simulink model "cv_model"  (R2023a)
settings: Solver=ode23t  StartTime=0  StopTime=400  FixedStep=0.0005  MaxStep=.01  RelTol=1e-4
model workspace (MAT data in the model file):
  test = 0
values from neighbouring files (symbols this model uses):
  A_cheb_09_1 = [-9.45889157397 1 0 0 0 0 0 0 0 -116.684730988 0 1 ... (81 elements, 9x9)]    [input_reflex_filters.mat]
  B_cheb_09_1 = [1 0 0 0 0 0 0 0 0]    [input_reflex_filters.mat]
  C_cheb_09_1 = [0 0 0 0 0 0 0 0 151338.279895]    [input_reflex_filters.mat]
libraries: SignalEditorBlockLib x4, simulink_extras x2
(part 1 of 3)
settings Model: ExtModeTrigMode=oneshot  Creator=samar  LastModifiedBy=Rich
settings SolverCC: AlgebraicLoopSolver=TrustRegion
settings DataIOCC: SaveFormat=Array  SignalLoggingSaveFormat=ModelDataLogs  ReturnWorkspaceOutputs=off  SignalLoggingName=sigsOut
settings OptimizationCC: BooleanDataType=off  InitFltsAndDblsToZero=on  LifeSpan=inf
settings DebuggingCC: ConsistencyChecking=warning  SaveWithParameterizedLinksMsg=none  UnderspecifiedInitializationDetection=Classic  MergeDetectMultiDrivingBlocksExec=none  SignalResolutionControl=TryResolveAllWithWarning  MultiTaskDSMMsg=warning  MultiTaskCondExecSysMsg=none  FcnCallInpInsideContextMsg=warning  SFUnexpectedBacktrackingDiag=warning  SFNoUnconditionalDefaultTransitionDiag=warning  SFExecutionAtInitializationDiag=none  ArithmeticOperatorsInVariantConditions=warning
settings HardwareCC: ProdBitPerPointer=32  ProdBitPerSizeT=32  ProdBitPerPtrDiffT=32  ProdLargestAtomicFloat=None  ProdIntDivRoundTo=Undefined  ProdEndianess=Unspecified  ProdWordSize=32  ProdHWDeviceType=32-bit Generic  TargetUnknown=on
settings ModelReferenceCC: EnableRefExpFcnMdlSchedulingChecks=on  PropagateSignalLabelsOutOfModel=off
settings SFSimCC: SimUseLocalCustomCode=off  CustomCodeUndefinedFunction=UseInterfaceOnly
settings RTWCC: TemplateMakefile=grt_unix.tmf  RTWUseLocalCustomCode=off  DLArmComputeVersion=19.05
settings CodeAppCC: StateflowObjectComments=on
settings GRTTargetCC: TargetFcnLib=ansi_tfl_tmw.mat  TargetLangStandard=C89/C90 (ANSI)  ModelReferenceCompliant=off  CombineOutputUpdateFcns=off  MatFileLogging=off  GRTInterface=on
settings ConfigComp: CovMetricSettings=dw  CovSaveCumulativeToWorkspaceVar=on  CovSaveSingleToWorkspaceVar=on  CovExternalEMLEnable=off  CovSFcnEnable=off

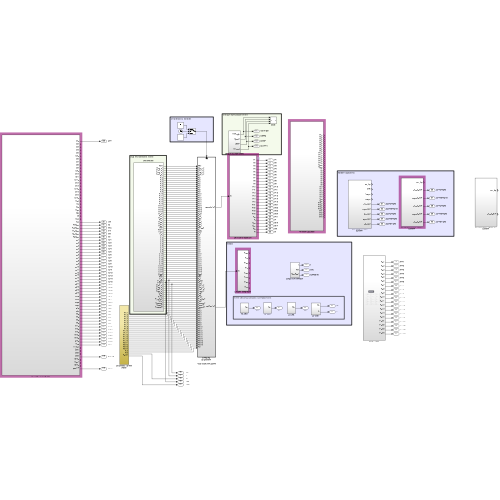
[thumbnail: Simulink's stored preview of the top-level diagram]
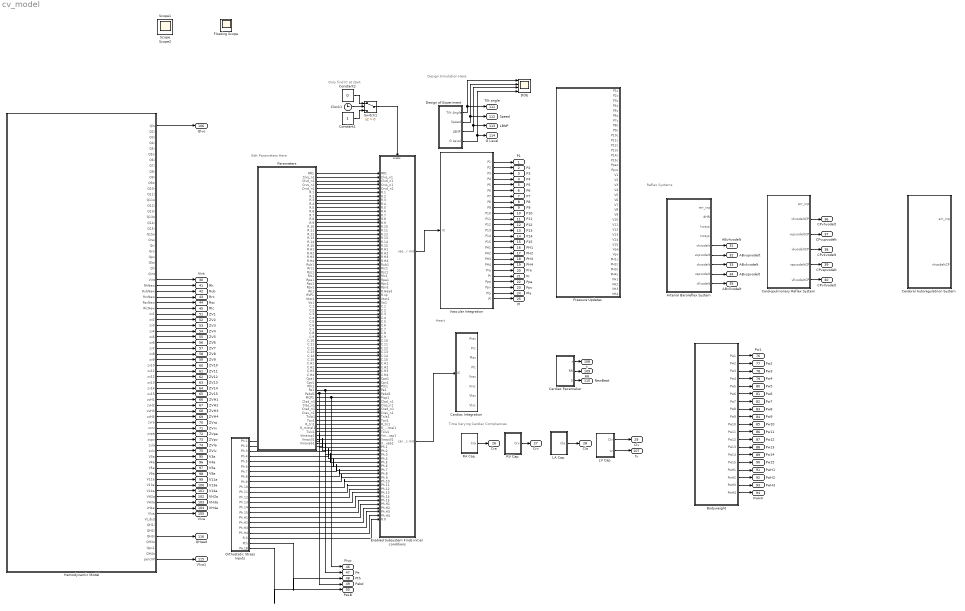
== system cv_model ==
  note: Design Simulation Here
  note: Edit Parameters Here
  note: Reflex Systems
  note: Heart
  note: Time Varying Cardiac Compliances
  note: Only find IC at start
  Arterial Baroreflex System : Subsystem
  Bodyweight : Subsystem
  Cardiac Integration : Subsystem
  Cardiac Pacemaker : Subsystem
  Cardiopulmonary Reflex System : Subsystem
  Cerebral Autoregulatrion System : Subsystem
  Clock1 : Clock
  Constant1 : Constant
  Constant2 : Constant  Value=0
  DOE : Scope  NumInputPorts=4
  Design of Experiment : Subsystem
  Enabled Subsystem Finds initial conditions : Subsystem  TreatAsAtomicUnit=on
  Hemodynamic Model : Subsystem
  LA Cap. : Subsystem
  LV Cap. : Subsystem
  Orthostatic Stress Inputs : Subsystem
  Parameters : Subsystem
  Pressure Updates : Subsystem
  RA Cap. : Subsystem
  RV Cap. : Subsystem
  Switch1 : Switch  Criteria=u2 > Threshold
  Vascular Integration : Subsystem
  P1 : Outport
  P2 : Outport  Port=2
  P3 : Outport  Port=3
  P4 : Outport  Port=4
  P5 : Outport  Port=5
  P6 : Outport  Port=6
  P7 : Outport  Port=7
  P8 : Outport  Port=8
  P9 : Outport  Port=9
  P10 : Outport  Port=10
  P11 : Outport  Port=11
  P12 : Outport  Port=12
  P13 : Outport  Port=13
  P14 : Outport  Port=14
  P15 : Outport  Port=15
  PH1 : Outport  Port=16
  PH2 : Outport  Port=17
  PH3 : Outport  Port=18
  PH4 : Outport  Port=19
  Pra : Outport  Port=20
  Pr : Outport  Port=21
  Ppa : Outport  Port=22
  Ppv : Outport  Port=23
  Pla : Outport  Port=24
  Pl : Outport  Port=25
  Cra : Outport  Port=26
  Crv : Outport  Port=27
  Cla : Outport  Port=28
  Clv : Outport  Port=29
  Vint : Outport  Port=30
  ABvhvodelt : Outport  Port=31
  ABvupvodelt : Outport  Port=32
  ABvkvodelt : Outport  Port=33
  ABvspvodelt : Outport  Port=34
  ABvllvodelt : Outport  Port=35
  CPvhvodelt : Outport  Port=36
  CPvupvodelt : Outport  Port=37
  CPvkvodelt : Outport  Port=38
  CPvspvodelt : Outport  Port=39
  CPvllvodelt : Outport  Port=40
  Rh : Outport  Port=41
  Rub : Outport  Port=42
  Rrc : Outport  Port=43
  Rsc : Outport  Port=44
  Rlc : Outport  Port=45
  Picp : Outport  Port=46
  Pe : Outport  Port=47
  Pth : Outport  Port=48
  Pabd : Outport  Port=49
  PeLB : Outport  Port=50
  ZV1 : Outport  Port=51
  ZV2 : Outport  Port=52
  ZV3 : Outport  Port=53
  ZV4 : Outport  Port=54
  ZV5 : Outport  Port=55
  ZV6 : Outport  Port=56
  ZV7 : Outport  Port=57
  ZV8 : Outport  Port=58
  ZV9 : Outport  Port=59
  ZV10 : Outport  Port=60
  ZV11 : Outport  Port=61
  ZV12 : Outport  Port=62
  ZV13 : Outport  Port=63
  ZV14 : Outport  Port=64
  ZV15 : Outport  Port=65
  ZVH1 : Outport  Port=66
  ZVH2 : Outport  Port=67
  ZVH3 : Outport  Port=68
  ZVH4 : Outport  Port=69
  ZVra : Outport  Port=70
  ZVrv : Outport  Port=71
  ZVpa : Outport  Port=72
  ZVpv : Outport  Port=73
  ZVla : Outport  Port=74
  ZVlv : Outport  Port=75
  Pw1 : Outport  Port=76
  Pw2 : Outport  Port=77
  Pw3 : Outport  Port=78
  Pw4 : Outport  Port=79
  Pw5 : Outport  Port=80
  Pw6 : Outport  Port=81
  Pw7 : Outport  Port=82
  Pw8 : Outport  Port=83
  Pw9 : Outport  Port=84
  Pw10 : Outport  Port=85
  Pw11 : Outport  Port=86
  Pw12 : Outport  Port=87
  Pw13 : Outport  Port=88
  Pw14 : Outport  Port=89
  Pw15 : Outport  Port=90
  PwH1 : Outport  Port=91
  PwH2 : Outport  Port=92
  PwH3 : Outport  Port=93
  PwH4 : Outport  Port=94
  V3a : Outport  Port=95
  V4a : Outport  Port=96
  V5a : Outport  Port=97
  V9a : Outport  Port=98
  V11a : Outport  Port=99
  V13a : Outport  Port=100
  V14a : Outport  Port=101
  VH2a : Outport  Port=102
  VH3a : Outport  Port=103
  VH4a : Outport  Port=104
  Vlva : Outport  Port=105
  Qlvo : Outport  Port=106
  tv : Outport  Port=107
  t : Outport  Port=108
  RR : Outport  Port=109
  NewBeat : Outport  Port=110
  Tilt angle : Outport  Port=111
  Speed : Outport  Port=112
  LBNP : Outport  Port=113
  G Level : Outport  Port=114
  Vlva1 : Outport  Port=115
  QHead : Outport  Port=116
  Floating Scope : Scope
  Scope : Scope
  Scope1 : Scope
  Scope2 : Scope
  wires:
  Enabled Subsystem Finds initial conditions/2(cardiac init) -> Cardiac Integration/1(IC)
  Enabled Subsystem Finds initial conditions/1(vascular init) -> Vascular Integration/1(IC)
  Constant2/1 -> Switch1/1
  Clock1/1 -> Switch1/2
  Constant1/1 -> Switch1/3
  Vascular Integration/25(Pl) -> Pl/1
  Vascular Integration/21(Pr) -> Pr/1
  Vascular Integration/22(Ppa) -> Ppa/1
  Vascular Integration/23(Ppv) -> Ppv/1
  Vascular Integration/1(P1) -> P1/1
  Vascular Integration/2(P2) -> P2/1
  Vascular Integration/3(P3) -> P3/1
  Vascular Integration/4(P4) -> P4/1
  Vascular Integration/5(P5) -> P5/1
  Vascular Integration/6(P6) -> P6/1
  Vascular Integration/7(P7) -> P7/1
  Vascular Integration/8(P8) -> P8/1
  Vascular Integration/9(P9) -> P9/1
  Vascular Integration/10(P10) -> P10/1
  Vascular Integration/11(P11) -> P11/1
  Vascular Integration/12(P12) -> P12/1
  Vascular Integration/13(P13) -> P13/1
  Vascular Integration/14(P14) -> P14/1
  Vascular Integration/15(P15) -> P15/1
  Arterial Baroreflex System/8(vspvodelt) -> ABvspvodelt/1
  Arterial Baroreflex System/6(vupvodelt) -> ABvupvodelt/1
  Cardiopulmonary Reflex System/5(vspvodeltCP) -> CPvspvodelt/1
  Cardiopulmonary Reflex System/4(vkvodeltCP) -> CPvkvodelt/1
  Cardiopulmonary Reflex System/6(vllvodeltCP) -> CPvllvodelt/1
  RA Cap./1(Cra) -> Cra/1
  LA Cap./1(Cla) -> Cla/1
  Cardiac Pacemaker/1(t) -> t/1
  LV Cap./1(Clv) -> Clv/1
  LV Cap./2(tv) -> tv/1
  RV Cap./1(Crv) -> Crv/1
  Vascular Integration/20(Pra) -> Pra/1
  Vascular Integration/24(Pla) -> Pla/1
  Arterial Baroreflex System/7(vkvodelt) -> ABvkvodelt/1
  Arterial Baroreflex System/9(vllvodelt) -> ABvllvodelt/1
  Cardiopulmonary Reflex System/3(vupvodeltCP) -> CPvupvodelt/1
  Orthostatic Stress Inputs/21(Pth) -> Pth/1
  Cardiac Pacemaker/2(RR) -> RR/1
  Cardiac Pacemaker/3(NewBeat) -> NewBeat/1
  Orthostatic Stress Inputs/22(Pe.LB) -> PeLB/1
  Hemodynamic Model/63(V11a) -> V11a/1
  Hemodynamic Model/33(RlcNew) -> Rlc/1
  Hemodynamic Model/62(V9a) -> V9a/1
  Hemodynamic Model/31(RrcNew) -> Rrc/1
  Hemodynamic Model/59(V3a) -> V3a/1
  Hemodynamic Model/32(RscNew) -> Rsc/1
  Hemodynamic Model/65(V14a) -> V14a/1
  Hemodynamic Model/69(Vlva) -> Vlva/1
  Hemodynamic Model/60(V4a) -> V4a/1
  Hemodynamic Model/30(RubNew) -> Rub/1
  Hemodynamic Model/61(V5a) -> V5a/1
  Design of Experiment/3(LBNP) -> DOE/3, LBNP/1
  Design of Experiment/1(Tilt Angle) -> Tilt angle/1, DOE/1
  Hemodynamic Model/28(Vint) -> Vint/1
  Design of Experiment/4(G Level) -> DOE/4, G Level/1
  Design of Experiment/2(Speed) -> DOE/2, Speed/1
  Parameters/59(Pabd1) -> Enabled Subsystem Finds initial conditions/59(Pabd1), Pabd/1
  Parameters/61(Clad_n1) -> Enabled Subsystem Finds initial conditions/61(Clad_n1)
  Parameters/62(Clas_n1) -> Enabled Subsystem Finds initial conditions/62(Clas_n1)
  Parameters/63(Crad_n1) -> Enabled Subsystem Finds initial conditions/63(Crad_n1)
  Parameters/64(Cras_n1) -> Enabled Subsystem Finds initial conditions/64(Cras_n1)
  Parameters/65(Tsla1) -> Enabled Subsystem Finds initial conditions/65(Tsla1)
  Parameters/66(Tav1) -> Enabled Subsystem Finds initial conditions/66(Tav1)
  Parameters/67(R_tri1) -> Enabled Subsystem Finds initial conditions/67(R_tri1)
  Parameters/68(R_mitral1) -> Enabled Subsystem Finds initial conditions/68(R_mitral1)
  Parameters/69(Tslv1) -> Enabled Subsystem Finds initial conditions/69(Tslv1)
  Parameters/70(Vmaxsp1) -> Enabled Subsystem Finds initial conditions/70(Vmaxsp1)
  Parameters/71(Vmaxll1) -> Enabled Subsystem Finds initial conditions/71(Vmaxll1)
  Parameters/72(Vmaxab1) -> Enabled Subsystem Finds initial conditions/72(Vmaxab1)
  Orthostatic Stress Inputs/1(Ph.1) -> Enabled Subsystem Finds initial conditions/73(Ph.1)
  Orthostatic Stress Inputs/2(Ph.2) -> Enabled Subsystem Finds initial conditions/74(Ph.2)
  Orthostatic Stress Inputs/3(Ph.3) -> Enabled Subsystem Finds initial conditions/75(Ph.3)
  Orthostatic Stress Inputs/4(Ph.4) -> Enabled Subsystem Finds initial conditions/76(Ph.4)
  Orthostatic Stress Inputs/5(Ph.5) -> Enabled Subsystem Finds initial conditions/77(Ph.5)
  Orthostatic Stress Inputs/6(Ph.6) -> Enabled Subsystem Finds initial conditions/78(Ph.6)
  Orthostatic Stress Inputs/7(Ph.7) -> Enabled Subsystem Finds initial conditions/79(Ph.7)
  Orthostatic Stress Inputs/8(Ph.8) -> Enabled Subsystem Finds initial conditions/80(Ph.8)
  Orthostatic Stress Inputs/9(Ph.9) -> Enabled Subsystem Finds initial conditions/81(Ph.9)
  Orthostatic Stress Inputs/10(Ph.10) -> Enabled Subsystem Finds initial conditions/82(Ph.10)
  Orthostatic Stress Inputs/11(Ph.11) -> Enabled Subsystem Finds initial conditions/83(Ph.11)
  Orthostatic Stress Inputs/12(Ph.12) -> Enabled Subsystem Finds initial conditions/84(Ph.12)
  Orthostatic Stress Inputs/13(Ph.13) -> Enabled Subsystem Finds initial conditions/85(Ph.13)
  Orthostatic Stress Inputs/14(Ph.14) -> Enabled Subsystem Finds initial conditions/86(Ph.14)
  Orthostatic Stress Inputs/15(Ph.15) -> Enabled Subsystem Finds initial conditions/87(Ph.15)
  Orthostatic Stress Inputs/20(R.0) -> Enabled Subsystem Finds initial conditions/92(R.0)
  Parameters/1(RR1) -> Enabled Subsystem Finds initial conditions/1(RR1)
  Parameters/2(Clvs_n1) -> Enabled Subsystem Finds initial conditions/2(Clvs_n1)
  Parameters/3(Clvd_n1) -> Enabled Subsystem Finds initial conditions/3(Clvd_n1)
  Parameters/4(Crvs_n1) -> Enabled Subsystem Finds initial conditions/4(Crvs_n1)
  Parameters/5(Crvd_n1) -> Enabled Subsystem Finds initial conditions/5(Crvd_n1)
  Parameters/6(R.1) -> Enabled Subsystem Finds initial conditions/6(R.1)
  Parameters/7(R.2) -> Enabled Subsystem Finds initial conditions/7(R.2)
  Parameters/8(R.3) -> Enabled Subsystem Finds initial conditions/8(R.3)
  Parameters/9(R.4) -> Enabled Subsystem Finds initial conditions/9(R.4)
  Parameters/10(R.5) -> Enabled Subsystem Finds initial conditions/10(R.5)
  Parameters/11(R.6) -> Enabled Subsystem Finds initial conditions/11(R.6)
  Parameters/12(R.7) -> Enabled Subsystem Finds initial conditions/12(R.7)
  Parameters/13(R.8) -> Enabled Subsystem Finds initial conditions/13(R.8)
  Parameters/14(R.9) -> Enabled Subsystem Finds initial conditions/14(R.9)
  Parameters/15(R.10) -> Enabled Subsystem Finds initial conditions/15(R.10)
  Parameters/16(R.11) -> Enabled Subsystem Finds initial conditions/16(R.11)
  Parameters/17(R.12) -> Enabled Subsystem Finds initial conditions/17(R.12)
  Parameters/18(R.13) -> Enabled Subsystem Finds initial conditions/18(R.13)
  Parameters/19(R.14) -> Enabled Subsystem Finds initial conditions/19(R.14)
  Parameters/20(R.15) -> Enabled Subsystem Finds initial conditions/20(R.15)
  Parameters/25(Rub1) -> Enabled Subsystem Finds initial conditions/25(Rub1)
  Parameters/26(Rrc1) -> Enabled Subsystem Finds initial conditions/26(Rrc1)
  Parameters/27(Rsc1) -> Enabled Subsystem Finds initial conditions/27(Rsc1)
  Parameters/28(Rlc1) -> Enabled Subsystem Finds initial conditions/28(Rlc1)
  Parameters/29(Rpa1) -> Enabled Subsystem Finds initial conditions/29(Rpa1)
  Parameters/30(Rpc1) -> Enabled Subsystem Finds initial conditions/30(Rpc1)
  Parameters/31(Rpv1) -> Enabled Subsystem Finds initial conditions/31(Rpv1)
  Parameters/34(Vtot1) -> Enabled Subsystem Finds initial conditions/34(Vtot1)
  Parameters/35(Vo1) -> Enabled Subsystem Finds initial conditions/35(Vo1)
  Parameters/36(C.1) -> Enabled Subsystem Finds initial conditions/36(C.1)
  Parameters/37(C.2) -> Enabled Subsystem Finds initial conditions/37(C.2)
  Parameters/38(C.3) -> Enabled Subsystem Finds initial conditions/38(C.3)
  Parameters/39(C.4) -> Enabled Subsystem Finds initial conditions/39(C.4)
  Parameters/40(C.5) -> Enabled Subsystem Finds initial conditions/40(C.5)
  Parameters/41(C.6) -> Enabled Subsystem Finds initial conditions/41(C.6)
  Parameters/42(C.7) -> Enabled Subsystem Finds initial conditions/42(C.7)
  Parameters/43(C.8) -> Enabled Subsystem Finds initial conditions/43(C.8)
  Parameters/44(C.9) -> Enabled Subsystem Finds initial conditions/44(C.9)
  Parameters/45(C.10) -> Enabled Subsystem Finds initial conditions/45(C.10)
  Parameters/46(C.11) -> Enabled Subsystem Finds initial conditions/46(C.11)
  Parameters/47(C.12) -> Enabled Subsystem Finds initial conditions/47(C.12)
  Parameters/48(C.13) -> Enabled Subsystem Finds initial conditions/48(C.13)
  Parameters/49(C.14) -> Enabled Subsystem Finds initial conditions/49(C.14)
  Parameters/50(C.15) -> Enabled Subsystem Finds initial conditions/50(C.15)
  Parameters/55(Cpa1) -> Enabled Subsystem Finds initial conditions/55(Cpa1)
  Parameters/56(Cpv1) -> Enabled Subsystem Finds initial conditions/56(Cpv1)
  Parameters/57(Pth1) -> Enabled Subsystem Finds initial conditions/57(Pth1)
  Hemodynamic Model/34(zv1) -> ZV1/1
  Hemodynamic Model/35(zv2) -> ZV2/1
  Hemodynamic Model/36(zv3) -> ZV3/1
  Hemodynamic Model/37(zv4) -> ZV4/1
  Hemodynamic Model/38(zv5) -> ZV5/1
  Hemodynamic Model/39(zv6) -> ZV6/1
  Hemodynamic Model/40(zv7) -> ZV7/1
  Hemodynamic Model/41(zv8) -> ZV8/1
  Hemodynamic Model/42(zv9) -> ZV9/1
  Hemodynamic Model/43(zv10) -> ZV10/1
  Hemodynamic Model/44(zv11) -> ZV11/1
  Hemodynamic Model/45(zv12) -> ZV12/1
  Hemodynamic Model/46(zv13) -> ZV13/1
  Hemodynamic Model/47(zv14) -> ZV14/1
  Hemodynamic Model/48(zv15) -> ZV15/1
  Hemodynamic Model/53(zvra) -> ZVra/1
  Hemodynamic Model/54(zvrv) -> ZVrv/1
  Hemodynamic Model/55(zvpa) -> ZVpa/1
  Hemodynamic Model/56(zvpv) -> ZVpv/1
  Hemodynamic Model/57(zvla) -> ZVla/1
  Hemodynamic Model/58(zvlv) -> ZVlv/1
  Hemodynamic Model/64(V13a) -> V13a/1
  Hemodynamic Model/1(Qlo) -> Qlvo/1
  Switch1/1 -> Enabled Subsystem Finds initial conditions/Enable
  Parameters/21(R.H1) -> Enabled Subsystem Finds initial conditions/21(R.H1)
  Parameters/22(R.H2) -> Enabled Subsystem Finds initial conditions/22(R.H2)
  Parameters/23(R.H3) -> Enabled Subsystem Finds initial conditions/23(R.H3)
  Parameters/24(R.H4) -> Enabled Subsystem Finds initial conditions/24(R.H4)
  Parameters/32(Rh1) -> Enabled Subsystem Finds initial conditions/32(R.Head)
  Parameters/33(RVP1) -> Enabled Subsystem Finds initial conditions/33(R.vp)
  Parameters/51(C.H1) -> Enabled Subsystem Finds initial conditions/51(C.H1)
  Parameters/52(C.H2) -> Enabled Subsystem Finds initial conditions/52(C.H2)
  Parameters/53(C.H3) -> Enabled Subsystem Finds initial conditions/53(C.H3)
  Parameters/54(C.H4) -> Enabled Subsystem Finds initial conditions/54(C.H4)
  Parameters/60(PICP1) -> Enabled Subsystem Finds initial conditions/60(Picp1), Picp/1
  Orthostatic Stress Inputs/16(Ph.H1) -> Enabled Subsystem Finds initial conditions/88(Ph.H1)
  Orthostatic Stress Inputs/17(Ph.H2) -> Enabled Subsystem Finds initial conditions/89(Ph.H2)
  Orthostatic Stress Inputs/18(Ph.H3) -> Enabled Subsystem Finds initial conditions/90(Ph.H3)
  Orthostatic Stress Inputs/19(Ph.H4) -> Enabled Subsystem Finds initial conditions/91(Ph.H4)
  Vascular Integration/16(PH1) -> PH1/1
  Vascular Integration/17(PH2) -> PH2/1
  Vascular Integration/18(PH3) -> PH3/1
  Vascular Integration/19(PH4) -> PH4/1
  Arterial Baroreflex System/5(vhvodelt) -> ABvhvodelt/1
  Cardiopulmonary Reflex System/2(vhvodeltCP) -> CPvhvodelt/1
  Hemodynamic Model/29(RhNew) -> Rh/1
  Hemodynamic Model/49(zvH1) -> ZVH1/1
  Hemodynamic Model/50(zvH2) -> ZVH2/1
  Hemodynamic Model/51(zvH3) -> ZVH3/1
  Hemodynamic Model/52(zvH4) -> ZVH4/1
  Hemodynamic Model/66(VH2a) -> VH2a/1
  Hemodynamic Model/67(VH3a) -> VH3a/1
  Hemodynamic Model/68(vH4a) -> VH4a/1
  Parameters/58(Pe1) -> Enabled Subsystem Finds initial conditions/58(Pe1), Pe/1
  Bodyweight/1(Pw1) -> Pw1/1
  Bodyweight/2(Pw2) -> Pw2/1
  Bodyweight/3(Pw3) -> Pw3/1
  Bodyweight/4(Pw4) -> Pw4/1
  Bodyweight/5(Pw5) -> Pw5/1
  Bodyweight/6(Pw6) -> Pw6/1
  Bodyweight/7(Pw7) -> Pw7/1
  Bodyweight/8(Pw8) -> Pw8/1
  Bodyweight/9(Pw9) -> Pw9/1
  Bodyweight/10(Pw10) -> Pw10/1
  Bodyweight/11(Pw11) -> Pw11/1
  Bodyweight/12(Pw12) -> Pw12/1
  Bodyweight/13(Pw13) -> Pw13/1
  Bodyweight/14(Pw14) -> Pw14/1
  Bodyweight/15(Pw15) -> Pw15/1
  Bodyweight/16(PwH1) -> PwH1/1
  Bodyweight/17(PwH2) -> PwH2/1
  Bodyweight/18(PwH3) -> PwH3/1
  Bodyweight/19(PwH4) -> PwH4/1
  Hemodynamic Model/77(percVP) -> Vlva1/1
  Hemodynamic Model/73(QH3i) -> QHead/1

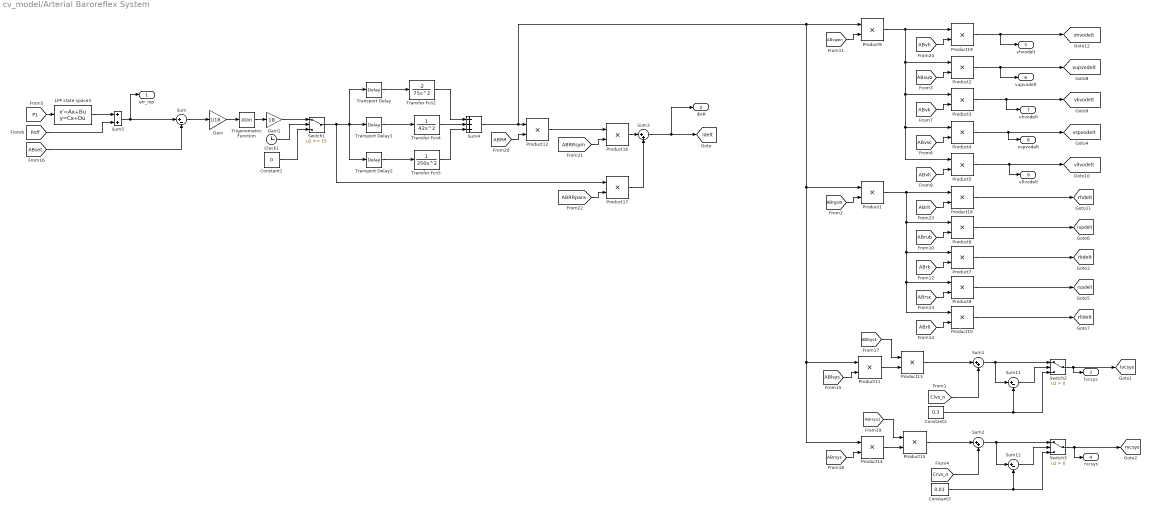
== system cv_model/Arterial Baroreflex System ==
  Clock1 : Clock
  Constant1 : Constant  Value=0
  Constant2 : Constant  Value=0.3
  Constant3 : Constant  Value=0.01
  Gain : Gain  Gain=1/18  SaturateOnIntegerOverflow=on  OutDataTypeStr=Inherit: Same as input  ParamDataTypeStr=Inherit: Same as input
  Gain1 : Gain  Gain=18  SaturateOnIntegerOverflow=on  OutDataTypeStr=Inherit: Same as input  ParamDataTypeStr=Inherit: Same as input
  LPF state space3 : StateSpace  A=A_cheb_09_1  B=B_cheb_09_1  C=C_cheb_09_1  D=0  InitialCondition=[0 0 0 0 0 0 0 0 91/C_cheb_09_1(9)]
  Product{1..19} (19 alike) : Product  Inputs=**  SaturateOnIntegerOverflow=on  OutDataTypeStr=Inherit: Same as first input
  Sum : Sum  Inputs=|+-  InputSameDT=on  SaturateOnIntegerOverflow=on  OutDataTypeStr=Inherit: Same as first input
  Sum1 : Sum  Inputs=|++  InputSameDT=on  SaturateOnIntegerOverflow=on  OutDataTypeStr=Inherit: Same as first input
  Sum11 : Sum  Inputs=|+-  InputSameDT=on  SaturateOnIntegerOverflow=on  OutDataTypeStr=Inherit: Same as first input
  Sum12 : Sum  Inputs=|+-  InputSameDT=on  SaturateOnIntegerOverflow=on  OutDataTypeStr=Inherit: Same as first input
  Sum2 : Sum  Inputs=|++  InputSameDT=on  SaturateOnIntegerOverflow=on  OutDataTypeStr=Inherit: Same as first input
  Sum3 : Sum  Inputs=|++  InputSameDT=on  SaturateOnIntegerOverflow=on  OutDataTypeStr=Inherit: Same as first input
  Sum4 : Sum  Inputs=+++  InputSameDT=on  SaturateOnIntegerOverflow=on  OutDataTypeStr=Inherit: Same as first input
  Sum5 : Sum  InputSameDT=on  SaturateOnIntegerOverflow=on  OutDataTypeStr=Inherit: Same as first input
  Switch1 : Switch  Threshold=15
  Switch2 : Switch  Criteria=u2 > Threshold
  Switch3 : Switch  Criteria=u2 > Threshold
  Transfer Fcn2 : TransferFcn  Numerator=-2  Denominator=[75 0 0]
  Transfer Fcn4 : TransferFcn  Numerator=1  Denominator=[42 0 0 ]
  Transfer Fcn5 : TransferFcn  Numerator=1  Denominator=[350 0 0 ]
  Transport Delay : TransportDelay  DelayTime=5
  Transport Delay1 : TransportDelay  DelayTime=2
  Transport Delay2 : TransportDelay  DelayTime=30  BufferSize=6144
  Trigonometric Function : Trigonometry  Operator=atan
  err_inp : Outport
  dHR : Outport  Port=2
  lvcsys : Outport  Port=3
  rvcsys : Outport  Port=4
  vhvodelt : Outport  Port=5
  vupvodelt : Outport  Port=6
  vkvodelt : Outport  Port=7
  vspvodelt : Outport  Port=8
  vllvodelt : Outport  Port=9
  tag scope: idelt=global, lvcsys=global, rhdelt=global, rkdelt=global, rlldelt=global, rspdelt=global, rupdelt=global, rvcsys=global, vhvodelt=global, vkvodelt=global, vllvodelt=global, vspvodelt=global, vupvodelt=global
  wires:
  Sum/1 -> Gain/1
  Product15/1 -> Sum2/1
  Product13/1 -> Sum1/1
  Sum1/1 -> Sum11/1, Switch2/1
  Product7/1 -> [rkdelt]
  Product4/1 -> [vspvodelt], vspvodelt/1
  [Crvs_n] -> Sum2/2
  [Clvs_n] -> Sum1/2
  Trigonometric Function/1 -> Gain1/1
  Product10/1 -> [rlldelt]
  Product6/1 -> [rupdelt]
  Product8/1 -> [rspdelt]
  Product2/1 -> vupvodelt/1, [vupvodelt]
  Product3/1 -> vkvodelt/1, [vkvodelt]
  Product5/1 -> vllvodelt/1, [vllvodelt]
  Product9/1 -> Product19/1, Product2/1, Product3/1, Product4/1, Product5/1
  Product1/1 -> Product18/1, Product6/1, Product7/1, Product8/1, Product10/1
  Sum4/1 -> Product12/1, Product9/1, Product14/1, Product11/1, Product1/1
  Gain1/1 -> Switch1/1
  Product16/1 -> Sum3/1
  Sum3/1 -> [idelt], dHR/1
  Product17/1 -> Sum3/2
  Clock1/1 -> Switch1/2
  Constant1/1 -> Switch1/3
  Switch1/1 -> Product17/1, Transport Delay1/1, Transport Delay/1, Transport Delay2/1
  Gain/1 -> Trigonometric Function/1
  Sum5/1 -> err_inp/1, Sum/1
  Sum11/1 -> Switch2/2
  Constant2/1 -> Switch2/3, Sum11/2
  Switch2/1 -> [lvcsys], lvcsys/1
  Sum2/1 -> Switch3/1, Sum12/1
  Sum12/1 -> Switch3/2
  Constant3/1 -> Switch3/3, Sum12/2
  Switch3/1 -> [rvcsys], rvcsys/1
  [P1] -> LPF state space3/1
  Transport Delay/1 -> Transfer Fcn2/1
  Transport Delay1/1 -> Transfer Fcn4/1
  Transport Delay2/1 -> Transfer Fcn5/1
  Transfer Fcn2/1 -> Sum4/1
  Transfer Fcn4/1 -> Sum4/2
  Transfer Fcn5/1 -> Sum4/3
  LPF state space3/1 -> Sum5/1
  [Poff] -> Sum5/2
  [ABset] -> Sum/2
  [ABvgain] -> Product9/2
  [ABrgain] -> Product1/2
  [ABvub] -> Product2/2
  [ABvk] -> Product3/2
  [ABvsc] -> Product4/2
  [ABvll] -> Product5/2
  [ABrub] -> Product6/2
  [ABrk] -> Product7/2
  [ABrsc] -> Product8/2
  [ABrll] -> Product10/2
  [ABlsys] -> Product11/2
  Product11/1 -> Product13/2
  [ABlsys1] -> Product13/1
  [ABrsys1] -> Product15/1
  [ABrsys] -> Product14/2
  Product14/1 -> Product15/2
  [ABRR] -> Product12/2
  [ABRRsym] -> Product16/2
  Product12/1 -> Product16/1
  [ABRRpara] -> Product17/2
  [ABrh] -> Product18/2
  Product18/1 -> [rhdelt]
  Product19/1 -> vhvodelt/1, [vhvodelt]
  [ABvh] -> Product19/2

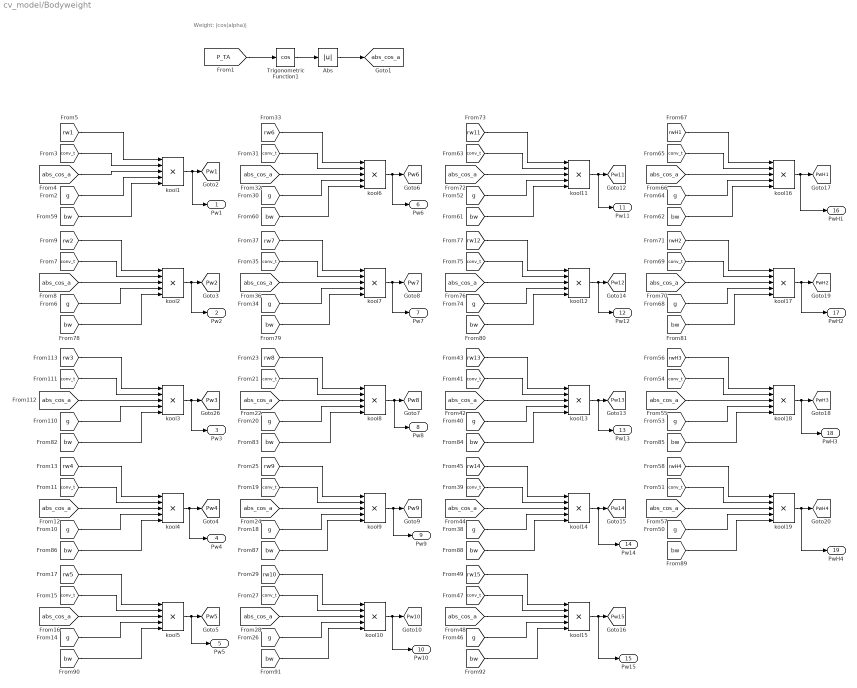
== system cv_model/Bodyweight ==
  note: Weight: |cos(alpha)|
  Abs : Abs  SaturateOnIntegerOverflow=off
  Trigonometric Function1 : Trigonometry  Operator=cos
  kool{1..19} (19 alike) : Product  Inputs=*****  InputSameDT=on  SaturateOnIntegerOverflow=on  OutDataTypeStr=Inherit: Same as first input
  Pw1 : Outport
  Pw2 : Outport  Port=2
  Pw3 : Outport  Port=3
  Pw4 : Outport  Port=4
  Pw5 : Outport  Port=5
  Pw6 : Outport  Port=6
  Pw7 : Outport  Port=7
  Pw8 : Outport  Port=8
  Pw9 : Outport  Port=9
  Pw10 : Outport  Port=10
  Pw11 : Outport  Port=11
  Pw12 : Outport  Port=12
  Pw13 : Outport  Port=13
  Pw14 : Outport  Port=14
  Pw15 : Outport  Port=15
  PwH1 : Outport  Port=16
  PwH2 : Outport  Port=17
  PwH3 : Outport  Port=18
  PwH4 : Outport  Port=19
  tag scope: Pw10=global, Pw11=global, Pw12=global, Pw13=global, Pw14=global, Pw15=global, Pw1=global, Pw2=global, Pw3=global, Pw4=global, Pw5=global, Pw6=global, Pw7=global, Pw8=global, Pw9=global, PwH1=global, PwH2=global, PwH3=global, PwH4=global, abs_cos_a=global
  wires:
  [abs_cos_a] -> kool3/3
  [conv_t] -> kool3/2
  kool3/1 -> Pw3/1, [Pw3]
  [g] -> kool3/4
  [P_TA] -> Trigonometric Function1/1
  Trigonometric Function1/1 -> Abs/1
  Abs/1 -> [abs_cos_a]
  [rw3] -> kool3/1
  [conv_t] -> kool1/2
  [abs_cos_a] -> kool1/3
  [rw1] -> kool1/1
  kool1/1 -> Pw1/1, [Pw1]
  [g] -> kool1/4
  [conv_t] -> kool2/2
  [abs_cos_a] -> kool2/3
  [rw2] -> kool2/1
  kool2/1 -> Pw2/1, [Pw2]
  [g] -> kool2/4
  [conv_t] -> kool4/2
  [abs_cos_a] -> kool4/3
  [rw4] -> kool4/1
  kool4/1 -> Pw4/1, [Pw4]
  [g] -> kool4/4
  [conv_t] -> kool5/2
  [abs_cos_a] -> kool5/3
  [rw5] -> kool5/1
  kool5/1 -> Pw5/1, [Pw5]
  [g] -> kool5/4
  [abs_cos_a] -> kool8/3
  kool8/1 -> Pw8/1, [Pw8]
  [conv_t] -> kool8/2
  [g] -> kool8/4
  kool7/1 -> Pw7/1, [Pw7]
  [conv_t] -> kool7/2
  [abs_cos_a] -> kool6/3
  [g] -> kool6/4
  [g] -> kool9/4
  kool6/1 -> Pw6/1, [Pw6]
  kool9/1 -> Pw9/1, [Pw9]
  [rw7] -> kool7/1
  [g] -> kool7/4
  [abs_cos_a] -> kool7/3
  [abs_cos_a] -> kool9/3
  [conv_t] -> kool9/2
  [conv_t] -> kool10/2
  [conv_t] -> kool6/2
  [rw9] -> kool9/1
  [abs_cos_a] -> kool10/3
  [g] -> kool10/4
  [rw6] -> kool6/1
  [rw10] -> kool10/1
  kool10/1 -> Pw10/1, [Pw10]
  [rw8] -> kool8/1
  kool13/1 -> Pw13/1, [Pw13]
  [conv_t] -> kool13/2
  [conv_t] -> kool16/2
  [g] -> kool13/4
  [rwH4] -> kool19/1
  [g] -> kool17/4
  [rwH1] -> kool16/1
  [conv_t] -> kool19/2
  [abs_cos_a] -> kool16/3
  kool19/1 -> PwH4/1, [PwH4]
  [conv_t] -> kool14/2
  [conv_t] -> kool15/2
  [conv_t] -> kool17/2
  [g] -> kool16/4
  [g] -> kool18/4
  [g] -> kool19/4
  [rwH3] -> kool18/1
  [rw15] -> kool15/1
  [abs_cos_a] -> kool13/3
  kool12/1 -> Pw12/1, [Pw12]
  kool17/1 -> PwH2/1, [PwH2]
  kool16/1 -> PwH1/1, [PwH1]
  [abs_cos_a] -> kool18/3
  [rwH2] -> kool17/1
  [conv_t] -> kool18/2
  [conv_t] -> kool12/2
  [abs_cos_a] -> kool12/3
  [g] -> kool12/4
  kool18/1 -> PwH3/1, [PwH3]
  [conv_t] -> kool11/2
  kool14/1 -> Pw14/1, [Pw14]
  [rw11] -> kool11/1
  [abs_cos_a] -> kool17/3
  [g] -> kool15/4
  [abs_cos_a] -> kool11/3
  [g] -> kool11/4
  kool11/1 -> Pw11/1, [Pw11]
  [g] -> kool14/4
  [rw12] -> kool12/1
  [abs_cos_a] -> kool19/3
  [abs_cos_a] -> kool14/3
  [rw14] -> kool14/1
  kool15/1 -> Pw15/1, [Pw15]
  [abs_cos_a] -> kool15/3
  [rw13] -> kool13/1
  [bw] -> kool1/5
  [bw] -> kool6/5
  [bw] -> kool11/5
  [bw] -> kool16/5
  [bw] -> kool2/5
  [bw] -> kool7/5
  [bw] -> kool12/5
  [bw] -> kool17/5
  [bw] -> kool3/5
  [bw] -> kool8/5
  [bw] -> kool13/5
  [bw] -> kool18/5
  [bw] -> kool4/5
  [bw] -> kool9/5
  [bw] -> kool14/5
  [bw] -> kool19/5
  [bw] -> kool5/5
  [bw] -> kool10/5
  [bw] -> kool15/5

== system cv_model/Cardiac Integration ==
  IC : Inport
  Demux1 : Demux
      settings: DisplayOption=none
  Integrator1 : Integrator  InitialConditionSource=external  InitialCondition=[220.105 68.078]
  Math Function1 : Math  Operator=reciprocal  SignedPower=on
  Math Function3 : Math  Operator=reciprocal  SignedPower=on
  Math Function4 : Math  Operator=reciprocal  SignedPower=on
  Mux2 : Mux
  Product : Product  Inputs=*/  SaturateOnIntegerOverflow=on  OutDataTypeStr=Inherit: Same as first input
  Product1 : Product  SaturateOnIntegerOverflow=on  OutDataTypeStr=Inherit: Same as first input
  Product2 : Product  SaturateOnIntegerOverflow=on  OutDataTypeStr=Inherit: Same as first input
  Product3 : Product  SaturateOnIntegerOverflow=on  OutDataTypeStr=Inherit: Same as first input
  Product4 : Product  Inputs=*/  SaturateOnIntegerOverflow=on  OutDataTypeStr=Inherit: Same as first input
  Sum{1..4} (4 alike) : Sum  InputSameDT=on  SaturateOnIntegerOverflow=on  OutDataTypeStr=Inherit: Same as first input
  Switch2 : Switch  Criteria=u2 > Threshold
  Prac : Outport
  Prc : Outport  Port=2
  Plac : Outport  Port=3
  Plc : Outport  Port=4
  Vrac : Outport  Port=5
  Vrvc : Outport  Port=6
  Vlac : Outport  Port=7
  Vlvc : Outport  Port=8
  tag scope: Pl=global, Pla=global, Pr=global, Pra=global, Vl_dist=global, Vla=global, Vra=global, Vrv=global
  wires:
  Mux2/1 -> Integrator1/1
  [dVl] -> Mux2/1
  [dVr] -> Mux2/2
  Integrator1/1 -> Demux1/1
  [Crv] -> Math Function1/1
  Math Function1/1 -> Product1/2
  Demux1/2 -> Product1/1, [Vrv], Vrvc/1
  Product1/1 -> Sum1/1, Prc/1
  [Pth] -> Sum1/2
  Sum1/1 -> [Pr]
  [Pth] -> Sum2/2
  Sum2/1 -> [Pl]
  IC/1 -> Integrator1/2
  [dVla] -> Mux2/3
  [dVra] -> Mux2/4
  [Cla] -> Math Function3/1
  Math Function3/1 -> Product2/2
  Product2/1 -> Plac/1, Sum3/1
  [Pth] -> Sum3/2
  [Cra] -> Math Function4/1
  Math Function4/1 -> Product3/2
  Product3/1 -> Sum4/1, Prac/1
  [Pth] -> Sum4/2
  Sum4/1 -> [Pra]
  Demux1/4 -> [Vra], Vrac/1, Product3/1
  [Clv] -> Switch2/1
  [ZVlv] -> Product4/1
  [Pcol] -> Product4/2
  Switch2/1 -> Product/2
  Product4/1 -> Switch2/3
  Product/1 -> Plc/1, Sum2/1
  Sum3/1 -> [Pla]
  Demux1/1 -> Switch2/2, Product/1, [Vl_dist], Vlvc/1
  Demux1/3 -> [Vla], Vlac/1, Product2/1

== system cv_model/Cardiac Pacemaker ==
  note: New Beat Logic
  note: Define New RR Interval
  note: Define m(n) = 1/I(n) = 1/(I0 + dI)
  Clock1 : Clock
  Clock2 : Clock
  Constant : Constant  Value=60
  Constant1 : Constant
  Constant2 : Constant  Value=0
  Constant4 : Constant  Value=0
  Divide : Product  Inputs=*/
  Gain1 : Gain  Gain=0.001
  Gain2 : Gain  Gain=0.2
  Gain3 : Gain  Gain=1.5
  Gain4 : Gain  Gain=0.001
  HRVisual : Scope
  Integrator : Integrator  ExternalReset=level  InitialConditionSource=external
  Logical Operator1 : Logic  Inputs=3  OutDataTypeStr=boolean
  Math Function2 : Math  Operator=reciprocal  SignedPower=on
  Memory1 : Memory  InitialCondition=-0.12*sqrt(6/7)-6/7  InheritSampleTime=on
  Memory2 : Memory  InheritSampleTime=on
  Memory3 : Memory  InitialCondition=-0.12*sqrt(6/7)  InheritSampleTime=on
  Memory4 : Memory  InheritSampleTime=on
  Relational Operator : RelationalOperator  OutDataTypeStr=boolean  InputSameDT=off
  Relational Operator1 : RelationalOperator  OutDataTypeStr=boolean  InputSameDT=off
  Relational Operator2 : RelationalOperator  OutDataTypeStr=boolean  InputSameDT=off
  Relational Operator3 : RelationalOperator  Operator=<  OutDataTypeStr=float('double')  InputSameDT=off
  Scope1 : Scope
  Sum1 : Sum  Inputs=+-  InputSameDT=on  SaturateOnIntegerOverflow=on  OutDataTypeStr=Inherit: Same as first input
  Sum11 : Sum  Inputs=+-  InputSameDT=on  SaturateOnIntegerOverflow=on  OutDataTypeStr=Inherit: Same as first input
  Sum2 : Sum  InputSameDT=on  SaturateOnIntegerOverflow=on  OutDataTypeStr=Inherit: Same as first input
  Sum3 : Sum  Inputs=+-  InputSameDT=on  SaturateOnIntegerOverflow=on  OutDataTypeStr=Inherit: Same as first input
  Switch1 : Switch  Threshold=0.5
  Switch2 : Switch  Criteria=u2 > Threshold
  Switch4 : Switch  Criteria=u2 > Threshold  Threshold=0.5
  mult1 : Product  Inputs=*/
  t : Outport
  RR : Outport  Port=2
  NewBeat : Outport  Port=3
  tag scope: NewBeat=global, RR=global, m=global, t=global
  wires:
  Switch4/1 -> Memory3/1, Sum1/1, Sum3/2
  Memory3/1 -> Switch4/3, Switch1/1
  Clock1/1 -> Switch4/1, Sum3/1
  [m] -> Integrator/1
  Integrator/1 -> Relational Operator/1, Sum11/1, Memory4/1
  Relational Operator/1 -> Logical Operator1/1
  Constant1/1 -> Relational Operator/2
  [RR0] -> Sum2/1
  [idelt] -> Sum2/2
  Sum2/1 -> Gain1/1
  Gain1/1 -> Math Function2/1
  Math Function2/1 -> [m]
  Logical Operator1/1 -> Integrator/2
  Relational Operator1/1 -> Logical Operator1/2
  Switch1/1 -> Memory1/1, Sum1/2
  Memory1/1 -> Switch1/3
  Sum1/1 -> [RR], Divide/2, RR/1
  Clock2/1 -> Switch2/2
  mult1/1 -> Switch2/3
  [Tav0] -> mult1/1
  Constant2/1 -> Switch2/1
  Switch2/1 -> Integrator/3
  Sum3/1 -> [t], t/1
  [t] -> Relational Operator1/1
  [RR] -> Gain2/1
  Gain2/1 -> Relational Operator1/2
  Relational Operator2/1 -> Logical Operator1/3
  [Tslv] -> Gain3/1
  Gain3/1 -> Relational Operator2/2
  [tv] -> Relational Operator2/1
  Memory4/1 -> Sum11/2
  Sum11/1 -> Relational Operator3/1
  Relational Operator3/1 -> Memory2/1
  Constant4/1 -> Relational Operator3/2
  [NewBeat] -> Switch1/2, Switch4/2
  Memory2/1 -> NewBeat/1, Scope1/1, [NewBeat]
  Constant/1 -> Divide/1
  Divide/1 -> HRVisual/1
  Gain4/1 -> mult1/2
  [RR0] -> Gain4/1

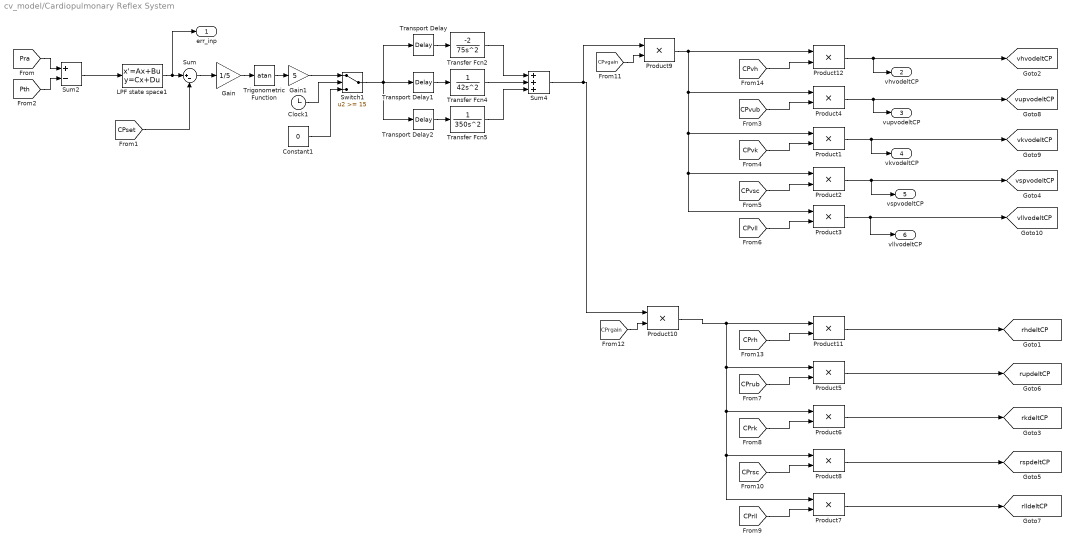
== system cv_model/Cardiopulmonary Reflex System ==
  Clock1 : Clock
  Constant1 : Constant  Value=0
  Gain : Gain  Gain=1/5  SaturateOnIntegerOverflow=on  OutDataTypeStr=Inherit: Same as input  ParamDataTypeStr=Inherit: Same as input
  Gain1 : Gain  Gain=5  SaturateOnIntegerOverflow=on  OutDataTypeStr=Inherit: Same as input  ParamDataTypeStr=Inherit: Same as input
  LPF state space1 : StateSpace  A=A_cheb_09_1  B=B_cheb_09_1  C=C_cheb_09_1  D=0  InitialCondition=[0 0 0 0 0 0 0 0 8.3/C_cheb_09_1(9)]
  Product{1..12} (12 alike) : Product  Inputs=**  SaturateOnIntegerOverflow=on  OutDataTypeStr=Inherit: Same as first input
  Sum : Sum  Inputs=|+-  InputSameDT=on  SaturateOnIntegerOverflow=on  OutDataTypeStr=Inherit: Same as first input
  Sum2 : Sum  Inputs=+-  InputSameDT=on  SaturateOnIntegerOverflow=on  OutDataTypeStr=Inherit: Same as first input
  Sum4 : Sum  Inputs=+++  InputSameDT=on  SaturateOnIntegerOverflow=on  OutDataTypeStr=Inherit: Same as first input
  Switch1 : Switch  Threshold=15
  Transfer Fcn2 : TransferFcn  Numerator=-2  Denominator=[75 0 0]
  Transfer Fcn4 : TransferFcn  Numerator=1  Denominator=[42 0 0 ]
  Transfer Fcn5 : TransferFcn  Numerator=1  Denominator=[350 0 0 ]
  Transport Delay : TransportDelay  DelayTime=5
  Transport Delay1 : TransportDelay  DelayTime=2
  Transport Delay2 : TransportDelay  DelayTime=30  BufferSize=6144
  Trigonometric Function : Trigonometry  Operator=atan
  err_inp : Outport
  vhvodeltCP : Outport  Port=2
  vupvodeltCP : Outport  Port=3
  vkvodeltCP : Outport  Port=4
  vspvodeltCP : Outport  Port=5
  vllvodeltCP : Outport  Port=6
  tag scope: rhdeltCP=global, rkdeltCP=global, rlldeltCP=global, rspdeltCP=global, rupdeltCP=global, vhvodeltCP=global, vkvodeltCP=global, vllvodeltCP=global, vspvodeltCP=global, vupvodeltCP=global
  wires:
  Sum/1 -> Gain/1
  [CPset] -> Sum/2
  Gain/1 -> Trigonometric Function/1
  Trigonometric Function/1 -> Gain1/1
  Product6/1 -> [rkdeltCP]
  Product2/1 -> [vspvodeltCP], vspvodeltCP/1
  Product7/1 -> [rlldeltCP]
  Product5/1 -> [rupdeltCP]
  Product8/1 -> [rspdeltCP]
  Product4/1 -> [vupvodeltCP], vupvodeltCP/1
  Product1/1 -> [vkvodeltCP], vkvodeltCP/1
  Product3/1 -> [vllvodeltCP], vllvodeltCP/1
  Product9/1 -> Product12/1, Product4/1, Product1/1, Product3/1, Product2/1
  [Pra] -> Sum2/1
  Gain1/1 -> Switch1/1
  Clock1/1 -> Switch1/2
  Constant1/1 -> Switch1/3
  [Pth] -> Sum2/2
  Sum2/1 -> LPF state space1/1
  LPF state space1/1 -> err_inp/1, Sum/1
  Switch1/1 -> Transport Delay1/1, Transport Delay2/1, Transport Delay/1
  Transfer Fcn5/1 -> Sum4/3
  Transfer Fcn4/1 -> Sum4/2
  Transfer Fcn2/1 -> Sum4/1
  Transport Delay2/1 -> Transfer Fcn5/1
  Transport Delay1/1 -> Transfer Fcn4/1
  Transport Delay/1 -> Transfer Fcn2/1
  Sum4/1 -> Product10/1, Product9/1
  [CPvub] -> Product4/2
  [CPvk] -> Product1/2
  [CPvsc] -> Product2/2
  [CPvll] -> Product3/2
  [CPrub] -> Product5/2
  [CPrk] -> Product6/2
  [CPrll] -> Product7/2
  [CPrsc] -> Product8/2
  [CPvgain] -> Product9/2
  [CPrgain] -> Product10/2
  [CPrh] -> Product11/2
  Product10/1 -> Product11/1, Product5/1, Product6/1, Product7/1, Product8/1
  Product11/1 -> [rhdeltCP]
  Product12/1 -> [vhvodeltCP], vhvodeltCP/1
  [CPvh] -> Product12/2

== system cv_model/Cerebral Autoregulatrion System ==
  Clock1 : Clock
  Constant1 : Constant  Value=0
  Gain : Gain  Gain=1/36  SaturateOnIntegerOverflow=on  OutDataTypeStr=Inherit: Same as input  ParamDataTypeStr=Inherit: Same as input
  Gain1 : Gain  Gain=36  SaturateOnIntegerOverflow=on  OutDataTypeStr=Inherit: Same as input  ParamDataTypeStr=Inherit: Same as input
  LPF state space1 : StateSpace  A=A_cheb_09_1  B=B_cheb_09_1  C=C_cheb_09_1  D=0  InitialCondition=[0 0 0 0 0 0 0 0 8.3/C_cheb_09_1(9)]
  Product{9..12} (4 alike) : Product  Inputs=**  SaturateOnIntegerOverflow=on  OutDataTypeStr=Inherit: Same as first input
  Scope : Scope  NumInputPorts=2
  Sum : Sum  Inputs=|+-  InputSameDT=on  SaturateOnIntegerOverflow=on  OutDataTypeStr=Inherit: Same as first input
  Sum2 : Sum  Inputs=+-  InputSameDT=on  SaturateOnIntegerOverflow=on  OutDataTypeStr=Inherit: Same as first input
  Sum4 : Sum  Inputs=+++  InputSameDT=on  SaturateOnIntegerOverflow=on  OutDataTypeStr=Inherit: Same as first input
  Switch1 : Switch  Threshold=15
  Transfer Fcn2 : TransferFcn  Numerator=-2  Denominator=[75 0 0]
  Transfer Fcn4 : TransferFcn  Numerator=1  Denominator=[42 0 0 ]
  Transfer Fcn5 : TransferFcn  Numerator=1  Denominator=[350 0 0 ]
  Transport Delay : TransportDelay  DelayTime=5
  Transport Delay1 : TransportDelay  DelayTime=2
  Transport Delay2 : TransportDelay  DelayTime=30  BufferSize=6144
  Trigonometric Function : Trigonometry  Operator=atan
  err_inp : Outport
  vhvodeltCP : Outport  Port=2
  wires:
  Sum/1 -> Gain/1
  [CBFset] -> Sum/2
  Gain/1 -> Trigonometric Function/1
  Trigonometric Function/1 -> Gain1/1
  Product9/1 -> Product12/1
  [PH2] -> Sum2/1
  Gain1/1 -> Switch1/1
  Clock1/1 -> Switch1/2
  Constant1/1 -> Switch1/3
  [ICP] -> Sum2/2
  Sum2/1 -> Scope/2, LPF state space1/1
  LPF state space1/1 -> err_inp/1, Sum/1
  Switch1/1 -> Transport Delay1/1, Transport Delay2/1, Transport Delay/1
  Transfer Fcn5/1 -> Sum4/3
  Transfer Fcn4/1 -> Sum4/2
  Transfer Fcn2/1 -> Sum4/1
  Transport Delay2/1 -> Transfer Fcn5/1
  Transport Delay1/1 -> Transfer Fcn4/1
  Transport Delay/1 -> Transfer Fcn2/1
  [CPvgain] -> Product9/2
  [CPrgain] -> Product10/2
  [CPrh] -> Product11/2
  Product10/1 -> Product11/1
  Product11/1 -> ?
  Product12/1 -> vhvodeltCP/1
  [CPvh] -> Product12/2
  Sum4/1 -> Scope/1

== system cv_model/Design of Experiment ==
  Centrifugation (RPM) : SignalEditorBlockLib/Signal Editor  FileName=doe_src.mat  ActiveScenario=x20RPM  ActiveSignal=RPM  IsBus=off  OutputBusObjectStr=Bus: BusObject  SampleTime=0  ZeroCross=off  OutputAfterFinalValue=Holding final value  Unit=inherit  PreserveSignalName=on  ApplySigPropsToAllScenarios=on
  Constant : Constant
  Gravity Level (g) : SignalEditorBlockLib/Signal Editor  FileName=doe_glevel.mat  ActiveScenario=Earth  ActiveSignal=G Level  IsBus=off  OutputBusObjectStr=Bus: BusObject  SampleTime=0  ZeroCross=off  OutputAfterFinalValue=Holding final value  Unit=inherit  PreserveSignalName=on  ApplySigPropsToAllScenarios=on
  LBNP (mmHg) : SignalEditorBlockLib/Signal Editor  FileName=doe_lbnp.mat  ActiveScenario=No_LBNP  ActiveSignal=LBNP Pressure  IsBus=off  OutputBusObjectStr=Bus: BusObject  SampleTime=0  ZeroCross=off  OutputAfterFinalValue=Holding final value  Unit=inherit  PreserveSignalName=on  ApplySigPropsToAllScenarios=on
  Switch Block : Subsystem
  Tilt (degrees) : SignalEditorBlockLib/Signal Editor  FileName=doe_tilt.mat  ActiveScenario=x90degree_Sustained  ActiveSignal=Tilt Angle  IsBus=off  OutputBusObjectStr=Bus: BusObject  SampleTime=0  ZeroCross=off  OutputAfterFinalValue=Holding final value  Unit=inherit  PreserveSignalName=on  ApplySigPropsToAllScenarios=on
  Toggle Switch : ToggleSwitchBlock  LabelPosition=Hide
      settings: Values={{'Centrifugation', 'Tilt'}, [0 1]}
  Toggle Switch1 : ToggleSwitchBlock
      settings: Values={{'Off', 'Body Weight'}, [0 1]}
  to rad : Gain  Gain=2*pi/360  SaturateOnIntegerOverflow=on  OutDataTypeStr=Inherit: Same as input  ParamDataTypeStr=Inherit: Same as input
  to rad/s : Gain  Gain=2*pi/60  SaturateOnIntegerOverflow=on  OutDataTypeStr=Inherit: Same as input  ParamDataTypeStr=Inherit: Same as input
  Tilt Angle : Outport
  Speed : Outport  Port=2
  LBNP : Outport  Port=3
  G Level : Outport  Port=4
  tag scope: G_LEVEL=global, P_LNBP=global, P_TA=global, W_RADS=global, bw=global
  wires:
  Tilt (degrees)/1 -> to rad/1
  LBNP (mmHg)/1 -> LBNP/1, [P_LNBP]
  Gravity Level (g)/1 -> [G_LEVEL], G Level/1
  Centrifugation (RPM)/1 -> to rad/s/1
  to rad/1 -> Switch Block/1(In1)
  to rad/s/1 -> Switch Block/2(In2)
  Switch Block/1(Tilt Angle) -> Tilt Angle/1, [P_TA]
  Switch Block/2(Speed) -> Speed/1, [W_RADS]
  Constant/1 -> [bw]

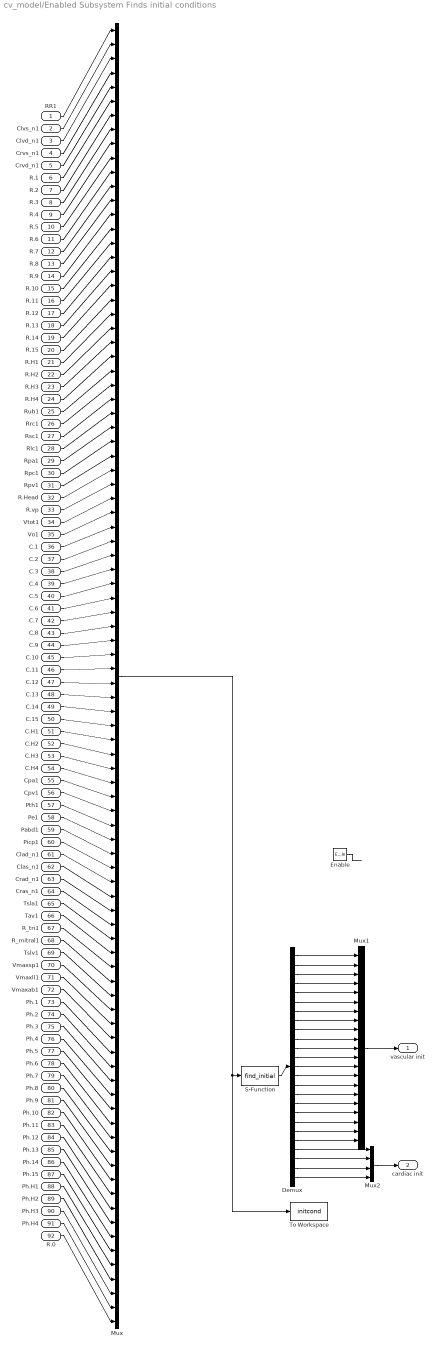
== system cv_model/Enabled Subsystem Finds initial conditions ==
  RR1 : Inport
  Clvs_n1 : Inport  Port=2
  Clvd_n1 : Inport  Port=3
  Crvs_n1 : Inport  Port=4
  Crvd_n1 : Inport  Port=5
  R.1 : Inport  Port=6
  R.2 : Inport  Port=7
  R.3 : Inport  Port=8
  R.4 : Inport  Port=9
  R.5 : Inport  Port=10
  R.6 : Inport  Port=11
  R.7 : Inport  Port=12
  R.8 : Inport  Port=13
  R.9 : Inport  Port=14
  R.10 : Inport  Port=15
  R.11 : Inport  Port=16
  R.12 : Inport  Port=17
  R.13 : Inport  Port=18
  R.14 : Inport  Port=19
  R.15 : Inport  Port=20
  R.H1 : Inport  Port=21
  R.H2 : Inport  Port=22
  R.H3 : Inport  Port=23
  R.H4 : Inport  Port=24
  Rub1 : Inport  Port=25
  Rrc1 : Inport  Port=26
  Rsc1 : Inport  Port=27
  Rlc1 : Inport  Port=28
  Rpa1 : Inport  Port=29
  Rpc1 : Inport  Port=30
  Rpv1 : Inport  Port=31
  R.Head : Inport  Port=32
  R.vp : Inport  Port=33
  Vtot1 : Inport  Port=34
  Vo1 : Inport  Port=35
  C.1 : Inport  Port=36
  C.2 : Inport  Port=37
  C.3 : Inport  Port=38
  C.4 : Inport  Port=39
  C.5 : Inport  Port=40
  C.6 : Inport  Port=41
  C.7 : Inport  Port=42
  C.8 : Inport  Port=43
  C.9 : Inport  Port=44
  C.10 : Inport  Port=45
  C.11 : Inport  Port=46
  C.12 : Inport  Port=47
  C.13 : Inport  Port=48
  C.14 : Inport  Port=49
  C.15 : Inport  Port=50
  C.H1 : Inport  Port=51
  C.H2 : Inport  Port=52
  C.H3 : Inport  Port=53
  C.H4 : Inport  Port=54
  Cpa1 : Inport  Port=55
  Cpv1 : Inport  Port=56
  Pth1 : Inport  Port=57
  Pe1 : Inport  Port=58
  Pabd1 : Inport  Port=59
  Picp1 : Inport  Port=60
  Clad_n1 : Inport  Port=61
  Clas_n1 : Inport  Port=62
  Crad_n1 : Inport  Port=63
  Cras_n1 : Inport  Port=64
  Tsla1 : Inport  Port=65
  Tav1 : Inport  Port=66
  R_tri1 : Inport  Port=67
  R_mitral1 : Inport  Port=68
  Tslv1 : Inport  Port=69
  Vmaxsp1 : Inport  Port=70
  Vmaxll1 : Inport  Port=71
  Vmaxab1 : Inport  Port=72
  Ph.1 : Inport  Port=73
  Ph.2 : Inport  Port=74
  Ph.3 : Inport  Port=75
  Ph.4 : Inport  Port=76
  Ph.5 : Inport  Port=77
  Ph.6 : Inport  Port=78
  Ph.7 : Inport  Port=79
  Ph.8 : Inport  Port=80
  Ph.9 : Inport  Port=81
  Ph.10 : Inport  Port=82
  Ph.11 : Inport  Port=83
  Ph.12 : Inport  Port=84
  Ph.13 : Inport  Port=85
  Ph.14 : Inport  Port=86
  Ph.15 : Inport  Port=87
  Ph.H1 : Inport  Port=88
  Ph.H2 : Inport  Port=89
  Ph.H3 : Inport  Port=90
  Ph.H4 : Inport  Port=91
  R.0 : Inport  Port=92
  Enable : EnablePort  ShowOutputPort=on
  Demux : Demux  Outputs=25
      settings: DisplayOption=none
  Mux : Mux  Inputs=92
  Mux1 : Mux  Inputs=21
  Mux2 : Mux
  S-Function : S-Function  FunctionName=find_initial  SFunctionDeploymentMode=off  EnableBusSupport=off
  To Workspace : ToWorkspace  VariableName=initcond  SampleTime=-1
  vascular init : Outport
  cardiac init : Outport  Port=2
  wires:
  Mux/1 -> S-Function/1, To Workspace/1
  S-Function/1 -> Demux/1
  Mux1/1 -> vascular init/1
  Mux2/1 -> cardiac init/1
  Demux/1 -> Mux1/1
  Demux/2 -> Mux1/2
  Demux/3 -> Mux1/3
  Demux/5 -> Mux1/5
  Demux/6 -> Mux1/6
  Demux/7 -> Mux1/7
  Demux/8 -> Mux1/8
  Demux/9 -> Mux1/9
  Demux/10 -> Mux1/10
  Demux/11 -> Mux1/11
  Demux/12 -> Mux1/12
  Demux/13 -> Mux1/13
  Demux/14 -> Mux1/14
  Demux/15 -> Mux1/15
  Demux/16 -> Mux1/16
  Demux/17 -> Mux1/17
  Enable/1 -> ?
  Demux/4 -> Mux1/4
  Demux/23 -> Mux2/2
  Demux/24 -> Mux2/3
  Demux/25 -> Mux2/4
  Demux/22 -> Mux2/1
  Demux/21 -> Mux1/21
  Demux/20 -> Mux1/20
  Demux/19 -> Mux1/19
  Demux/18 -> Mux1/18
  Rpc1/1 -> Mux/30
  Rpa1/1 -> Mux/29
  Rlc1/1 -> Mux/28
  Rsc1/1 -> Mux/27
  Rrc1/1 -> Mux/26
  Rub1/1 -> Mux/25
  R.H4/1 -> Mux/24
  R.H3/1 -> Mux/23
  R.H2/1 -> Mux/22
  R.H1/1 -> Mux/21
  R.15/1 -> Mux/20
  R.14/1 -> Mux/19
  R.13/1 -> Mux/18
  R.12/1 -> Mux/17
  R.11/1 -> Mux/16
  R.10/1 -> Mux/15
  R.9/1 -> Mux/14
  R.8/1 -> Mux/13
  R.7/1 -> Mux/12
  R.6/1 -> Mux/11
  R.5/1 -> Mux/10
  R.4/1 -> Mux/9
  R.3/1 -> Mux/8
  R.2/1 -> Mux/7
  R.1/1 -> Mux/6
  Crvd_n1/1 -> Mux/5
  Crvs_n1/1 -> Mux/4
  Clvd_n1/1 -> Mux/3
  Clvs_n1/1 -> Mux/2
  RR1/1 -> Mux/1
  Rpv1/1 -> Mux/31
  R.Head/1 -> Mux/32
  R.vp/1 -> Mux/33
  Vtot1/1 -> Mux/34
  Vo1/1 -> Mux/35
  C.1/1 -> Mux/36
  C.2/1 -> Mux/37
  C.3/1 -> Mux/38
  C.4/1 -> Mux/39
  C.5/1 -> Mux/40
  C.6/1 -> Mux/41
  C.7/1 -> Mux/42
  C.8/1 -> Mux/43
  C.9/1 -> Mux/44
  C.10/1 -> Mux/45
  C.11/1 -> Mux/46
  C.12/1 -> Mux/47
  C.13/1 -> Mux/48
  C.14/1 -> Mux/49
  C.15/1 -> Mux/50
  C.H1/1 -> Mux/51
  C.H2/1 -> Mux/52
  C.H3/1 -> Mux/53
  C.H4/1 -> Mux/54
  Cpa1/1 -> Mux/55
  Cpv1/1 -> Mux/56
  Pth1/1 -> Mux/57
  Pe1/1 -> Mux/58
  Pabd1/1 -> Mux/59
  Picp1/1 -> Mux/60
  Clad_n1/1 -> Mux/61
  Clas_n1/1 -> Mux/62
  Crad_n1/1 -> Mux/63
  Cras_n1/1 -> Mux/64
  Tsla1/1 -> Mux/65
  Tav1/1 -> Mux/66
  R_tri1/1 -> Mux/67
  R_mitral1/1 -> Mux/68
  Tslv1/1 -> Mux/69
  Vmaxsp1/1 -> Mux/70
  Vmaxll1/1 -> Mux/71
  Vmaxab1/1 -> Mux/72
  Ph.1/1 -> Mux/73
  Ph.2/1 -> Mux/74
  Ph.3/1 -> Mux/75
  Ph.4/1 -> Mux/76
  Ph.5/1 -> Mux/77
  Ph.6/1 -> Mux/78
  Ph.7/1 -> Mux/79
  Ph.8/1 -> Mux/80
  Ph.9/1 -> Mux/81
  Ph.10/1 -> Mux/82
  Ph.11/1 -> Mux/83
  Ph.12/1 -> Mux/84
  Ph.13/1 -> Mux/85
  Ph.14/1 -> Mux/86
  Ph.15/1 -> Mux/87
  Ph.H1/1 -> Mux/88
  Ph.H2/1 -> Mux/89
  Ph.H3/1 -> Mux/90
  Ph.H4/1 -> Mux/91
  R.0/1 -> Mux/92
